simulink model "third_1_debug"  (R2021b)
settings: Solver=FixedStepAuto  StartTime=0.0  StopTime=10  RelTol=1e-3
settings Model: Creator=fredric  LastModifiedBy=fredric

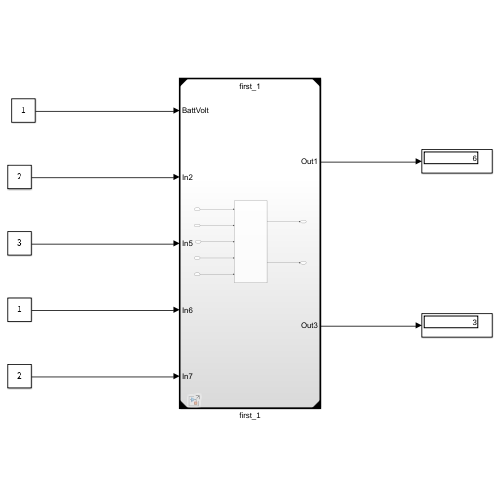
[thumbnail: Simulink's stored preview of the top-level diagram]
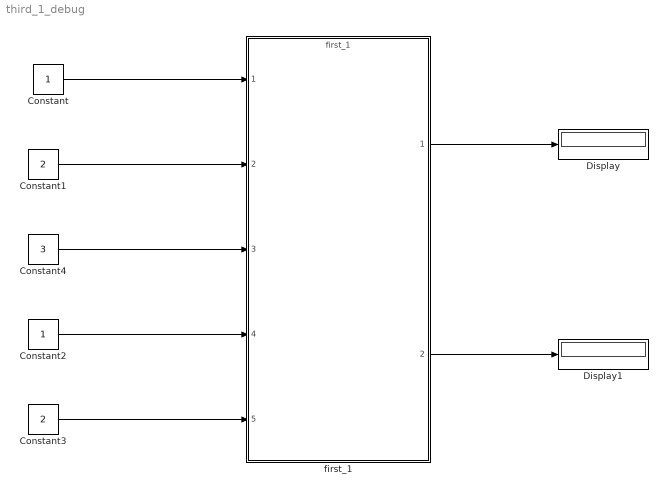
== system third_1_debug ==
  Constant : Constant
  Constant1 : Constant  Value=2
  Constant2 : Constant
  Constant3 : Constant  Value=2
  Constant4 : Constant  Value=3
  Display : Display
  Display1 : Display
  first_1 : ModelReference  ModelNameDialog=first_1  ModelReferenceVersion=1.4
  wires:
  Constant/1 -> first_1/1
  Constant1/1 -> first_1/2
  Constant2/1 -> first_1/4
  Constant4/1 -> first_1/3
  Constant3/1 -> first_1/5
  first_1/2 -> Display1/1
  first_1/1 -> Display/1
